simulink model "encoder_lcd"  (R2015a)
settings: Solver=ode45  StartTime=0.0  StopTime=10.0  RelTol=1e-3
libraries: legonxtlib x7
settings Model: Creator=Sondre  LastModifiedBy=Sondre

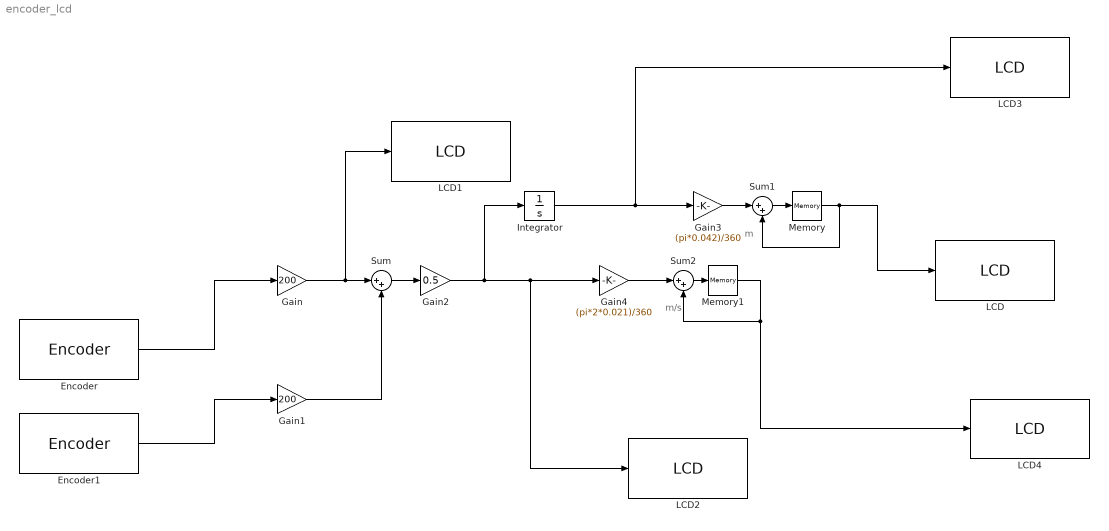
== system encoder_lcd ==
  note: m
  note: m/s
  Encoder : legonxtlib/Encoder  portNumber=A  opMode=Reset at each sample time  sampleTime=0.005  blockPlatform=LegoMindstormsNXT
  Encoder1 : legonxtlib/Encoder  portNumber=C  opMode=Reset at each sample time  sampleTime=0.005  blockPlatform=LegoMindstormsNXT
  Gain : Gain  Gain=200
  Gain1 : Gain  Gain=200
  Gain2 : Gain  Gain=0.5  OutDataTypeStr=double
  Gain3 : Gain  Gain=(pi*0.042)/360
  Gain4 : Gain  Gain=(pi*2*0.021)/360
  Integrator : Integrator
  LCD : legonxtlib/LCD  slcdStr=intmem  slcdLine=5  slcdFormat=Decimal  blockPlatform=LegoMindstormsNXT
  LCD1 : legonxtlib/LCD  slcdStr=a_raw  slcdLine=1  slcdFormat=Decimal  blockPlatform=LegoMindstormsNXT
  LCD2 : legonxtlib/LCD  slcdStr=2_raw  slcdLine=3  slcdFormat=Decimal  blockPlatform=LegoMindstormsNXT
  LCD3 : legonxtlib/LCD  slcdStr=int  slcdLine=4  slcdFormat=Decimal  blockPlatform=LegoMindstormsNXT
  LCD4 : legonxtlib/LCD  slcdStr=rawmem  slcdLine=6  slcdFormat=Decimal  blockPlatform=LegoMindstormsNXT
  Memory : Memory
  Memory1 : Memory
  Sum : Sum  Inputs=|++
  Sum1 : Sum  Inputs=|++
  Sum2 : Sum  Inputs=|++
  wires:
  Encoder1/1 -> Gain1/1
  Gain2/1 -> LCD2/1, Gain4/1, Integrator/1
  Sum/1 -> Gain2/1
  Encoder/1 -> Gain/1
  Memory/1 -> Sum1/2, LCD/1
  Gain3/1 -> Sum1/1
  Gain4/1 -> Sum2/1
  Sum1/1 -> Memory/1
  Sum2/1 -> Memory1/1
  Gain/1 -> LCD1/1, Sum/1
  Gain1/1 -> Sum/2
  Integrator/1 -> LCD3/1, Gain3/1
  Memory1/1 -> LCD4/1, Sum2/2
